simulink model "General_OL_model_NoFilters"  (R2020b)
settings: Solver=VariableStepAuto  StartTime=0.0  StopTime=10.0  RelTol=1e-3
undefined symbols (not defined in the file): Actuators, PAYLOAD
libraries: cstblocks x15, RCTblocks x1
settings Model: Creator=pa.iannelli  LastModifiedBy=f.sanfedino

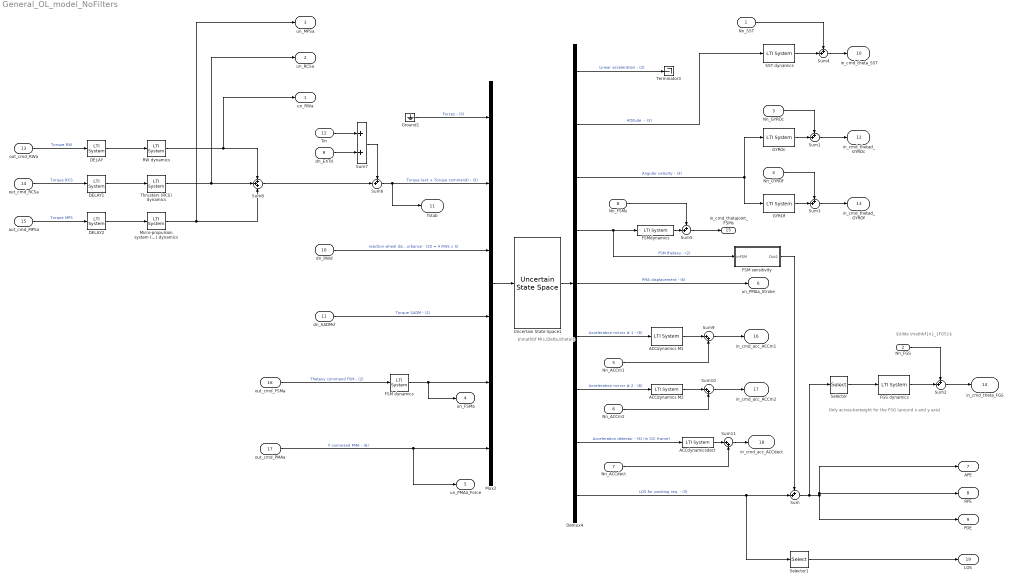
== system General_OL_model_NoFilters ==
  note: Only across-boresight for the FSG (around x and y axis)
  note: $\mathbf M(s,\Delta,\theta)$
  note: $\tilde \mathbf{n}_{FGS}$
  Nn_SST : Inport  PortDimensions=3
  Nn_FGS : Inport  Port=2  PortDimensions=2
  Nn_GYROc : Inport  Port=3  PortDimensions=3
  Nn_GYROf : Inport  Port=4  PortDimensions=3
  Nn_ACCm1 : Inport  Port=5  PortDimensions=6
  Nn_ACCm2 : Inport  Port=6  PortDimensions=6
  Nn_ACCdect : Inport  Port=7  PortDimensions=6
  Nn_FSMs : Inport  Port=8  PortDimensions=2
  dn_EXTd : Inport  Port=9  PortDimensions=3
  dn_RWd : Inport  Port=10
  dn_SADMd : Inport  Port=11
  Tin : Inport  Port=12  PortDimensions=3
  out_cmd_RWa : Inport  Port=13
  out_cmd_RCSa : Inport  Port=14
  out_cmd_MPSa : Inport  Port=15
  out_cmd_FSMa : Inport  Port=16
  out_cmd_PMAa : Inport  Port=17
  ACCdynamics M1 : cstblocks/LTI System  sys=Sensors.ACCm1.Dyn  IC=[]
  ACCdynamics M2 : cstblocks/LTI System  sys=Sensors.ACCm2.Dyn  IC=[]
  ACCdynamicsdect : cstblocks/LTI System  sys=Sensors.ACCdect.Dyn  IC=[]
  DELAY : cstblocks/LTI System  sys=Model.delay.Weight  IC=[]
  DELAY1 : cstblocks/LTI System  sys=Model.delay.Weight  IC=[]
  DELAY2 : cstblocks/LTI System  sys=Model.delay.Weight  IC=[]
  Demux4 : Demux  Outputs=[3,3,3,2,6,6,6,6,3]
  FGS dynamics : cstblocks/LTI System  sys=Sensors.FGS.Dyn  IC=[]
  FSM dynamics : cstblocks/LTI System  sys=ss(Actuators.FSM.Dyn)  IC=[]
  FSM sensitivity : Subsystem
  FSMdynamics : cstblocks/LTI System  sys=Sensors.FSM.Dyn  IC=[]
  GYROc : cstblocks/LTI System  sys=Sensors.GYROc.Dyn  IC=[]
  GYROf : cstblocks/LTI System  sys=Sensors.GYROf.Dyn  IC=[]
  Ground1 : Ground
  Micro-propulsion system (MPS) dynamics : cstblocks/LTI System  sys=Actuators.MPS.Dyn  IC=[]
  Mux2 : Mux  Inputs=[3,3,20,2,2,6]
  RW dynamics : cstblocks/LTI System  sys=Actuators.RW.Dyn  IC=[]
  SST dynamics : cstblocks/LTI System  sys=Sensors.SST.Dyn  IC=[]
  Selector : Selector  InputPortWidth=3  IndexOptions=Index vector (dialog)  Indices=[1 2]  OutputSizes=1
  Selector1 : Selector  InputPortWidth=3  IndexOptions=Index vector (dialog)  Indices=[1 2]  OutputSizes=1
  Sum{,1..6} (7 alike) : Sum  Inputs=++|
  Sum10 : Sum  Inputs=|++
  Sum11 : Sum  Inputs=|++
  Sum7 : Sum
  Sum8 : Sum  Inputs=+++
  Sum9 : Sum  Inputs=|++
  Terminator3 : Terminator
  Thrusters (RCS) dynamics : cstblocks/LTI System  sys=Actuators.RCS.Dyn  IC=[]
  Uncertain State Space1 : RCTblocks/Uncertain State Space  Tag=USS  SCDEnableBlockLinearizationSpecification=on  USystem=Gum_IOselected  UValue=[]  X0=[]  uX0=[]
      settings: SourceProductBaseCode=RC
  un_RWa : Outport
  un_RCSa : Outport  Port=2
  un_MPSa : Outport  Port=3
  un_FSMa : Outport  Port=4
  un_PMAa_Force : Outport  Port=5
  un_PMAa_Stroke : Outport  Port=6
  APE : Outport  Port=7
  RPE : Outport  Port=8
  PDE : Outport  Port=9
  in_cmd_theta_SST : Outport  Port=10
  Tstab : Outport  Port=11
  in_cmd_thetad_GYROc : Outport  Port=12
  in_cmd_thetad_GYROf : Outport  Port=13
  in_cmd_theta_FGS : Outport  Port=14
  in_cmd_thetaJoint_FSMs : Outport  Port=15
  in_cmd_acc_ACCm1 : Outport  Port=16
  in_cmd_acc_ACCm2 : Outport  Port=17
  in_cmd_acc_ACCdect : Outport  Port=18
  LOS : Outport  Port=19
  wires:
  Uncertain State Space1/1 -> Demux4/1
  Mux2/1 -> Uncertain State Space1/1
  Ground1/1 -> Mux2/1  "Forces - (3)"
  Sum6/1 -> Mux2/2, Tstab/1  "Torque (ext + Torque command) - (3)"
  dn_RWd/1 -> Mux2/3  "reaction wheel disturbance - (20 = 4 RWs x 5)"
  dn_SADMd/1 -> Mux2/4  "Torque SADM - (2)"
  out_cmd_FSMa/1 -> FSM dynamics/1  "Thetaxy command FSM - (2)"
  out_cmd_PMAa/1 -> un_PMAa_Force/1, Mux2/6  "F command PMA - (6)"
  Demux4/9 -> Selector1/1, Sum/2  "LOS for pointing req. - (3)"
  Demux4/1 -> Terminator3/1  "Linear acceleration - (3)"
  Demux4/3 -> GYROf/1, GYROc/1  "Angular velocity - (3)"
  Demux4/4 -> FSMdynamics/1, FSM sensitivity/1(inFSM)  "FSM thetaxy - (2)"
  Demux4/5 -> un_PMAa_Stroke/1  "PMA displacement - (6)"
  Demux4/6 -> ACCdynamics M1/1  "Acceleration mirror # 1 - (6)"
  Demux4/7 -> ACCdynamics M2/1  "Acceleration mirror # 2 - (6)"
  Demux4/8 -> ACCdynamicsdect/1  "Acceleration detector - (6) (in S/C frame)"
  Sum/1 -> Selector/1, APE/1, RPE/1, PDE/1
  Nn_SST/1 -> Sum4/1
  SST dynamics/1 -> Sum4/2
  GYROc/1 -> Sum1/2
  Sum1/1 -> in_cmd_thetad_GYROc/1
  out_cmd_RWa/1 -> DELAY/1  "Torque RW"
  DELAY/1 -> RW dynamics/1
  Sum8/1 -> Sum6/2
  Tin/1 -> Sum7/1
  dn_EXTd/1 -> Sum7/2
  Sum7/1 -> Sum6/1
  RW dynamics/1 -> un_RWa/1, Sum8/1
  DELAY1/1 -> Thrusters (RCS) dynamics/1
  DELAY2/1 -> Micro-propulsion system (MPS) dynamics/1
  out_cmd_RCSa/1 -> DELAY1/1  "Torque RCS"
  out_cmd_MPSa/1 -> DELAY2/1  "Torque MPS"
  Thrusters (RCS) dynamics/1 -> un_RCSa/1, Sum8/2
  Micro-propulsion system (MPS) dynamics/1 -> un_MPSa/1, Sum8/3
  Nn_ACCm1/1 -> Sum9/2
  Nn_ACCm2/1 -> Sum10/2
  Nn_ACCdect/1 -> Sum11/2
  Sum9/1 -> in_cmd_acc_ACCm1/1
  Sum10/1 -> in_cmd_acc_ACCm2/1
  Sum11/1 -> in_cmd_acc_ACCdect/1
  Nn_GYROc/1 -> Sum1/1
  Nn_GYROf/1 -> Sum3/1
  FGS dynamics/1 -> Sum2/2
  Sum2/1 -> in_cmd_theta_FGS/1
  Nn_FGS/1 -> Sum2/1
  Selector/1 -> FGS dynamics/1
  FSM dynamics/1 -> un_FSMa/1, Mux2/5
  GYROf/1 -> Sum3/2
  Sum5/1 -> in_cmd_thetaJoint_FSMs/1
  Sum3/1 -> in_cmd_thetad_GYROf/1
  Sum4/1 -> in_cmd_theta_SST/1
  Demux4/2 -> SST dynamics/1  "Attitude  - (3)"
  ACCdynamics M1/1 -> Sum9/1
  ACCdynamics M2/1 -> Sum10/1
  ACCdynamicsdect/1 -> Sum11/1
  Selector1/1 -> LOS/1
  FSM sensitivity/1(Out1) -> Sum/1
  FSMdynamics/1 -> Sum5/2
  Nn_FSMs/1 -> Sum5/1

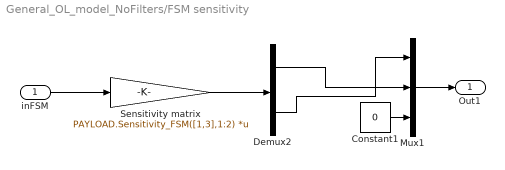
== system General_OL_model_NoFilters/FSM sensitivity ==
  inFSM : Inport
  Constant1 : Constant  Value=0
  Demux2 : Demux  Outputs=2
  Mux1 : Mux  Inputs=3
  Sensitivity matrix : Gain  Gain=PAYLOAD.Sensitivity_FSM([1,3],1:2)  Multiplication=Matrix(K*u) (u vector)
  Out1 : Outport
  wires:
  inFSM/1 -> Sensitivity matrix/1
  Constant1/1 -> Mux1/3
  Demux2/1 -> Mux1/2
  Sensitivity matrix/1 -> Demux2/1
  Mux1/1 -> Out1/1
  Demux2/2 -> Mux1/1
